simulink model "topcenterdown"  (Simulink 7.7)
settings: Solver=ode45  StartTime=0.0  StopTime=10.0  RelTol=1e-3
settings Model: Creator=Jx  LastModifiedBy=Jx

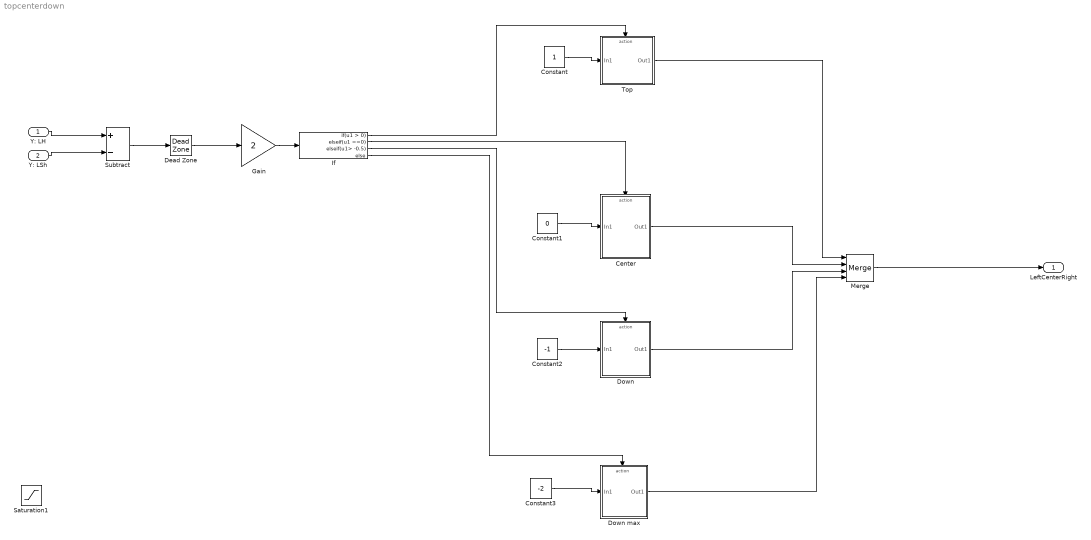
== system topcenterdown ==
  Y: LH : Inport
  Y: LSh : Inport  Port=2
  Center : Subsystem  TreatAsAtomicUnit=on
  Constant : Constant
  Constant1 : Constant  Value=0
  Constant2 : Constant  Value=-1
  Constant3 : Constant  Value=-2
  Dead Zone : DeadZone  LowerValue=-0.12  UpperValue=0.12  SaturateOnIntegerOverflow=on
  Down : Subsystem  TreatAsAtomicUnit=on
  Down max : Subsystem  TreatAsAtomicUnit=on
  Gain : Gain  Gain=2
  If : If  ElseIfExpressions=u1 ==0, u1> -0.5
  Merge : Merge  Inputs=4
  Saturation1 : Saturate  UpperLimit=1  LowerLimit=-1
  Subtract : Sum  Inputs=+-
  Top : Subsystem  TreatAsAtomicUnit=on
  LeftCenterRight : Outport
  wires:
  Y: LSh/1 -> Subtract/2
  Y: LH/1 -> Subtract/1
  Subtract/1 -> Dead Zone/1
  If/1 -> Top/Action
  If/2 -> Center/Action
  If/3 -> Down/Action
  If/4 -> Down max/Action
  Constant/1 -> Top/1(In1)
  Dead Zone/1 -> Gain/1
  Gain/1 -> If/1
  Constant1/1 -> Center/1(In1)
  Constant2/1 -> Down/1(In1)
  Constant3/1 -> Down max/1(In1)
  Center/1(Out1) -> Merge/2
  Down/1(Out1) -> Merge/3
  Down max/1(Out1) -> Merge/4
  Top/1(Out1) -> Merge/1
  Merge/1 -> LeftCenterRight/1

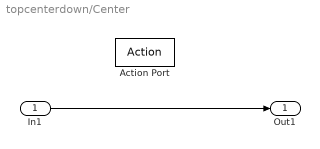
== system topcenterdown/Center ==
  In1 : Inport
  Action Port : ActionPort  ActionType=elseif
  Out1 : Outport
  wires:
  In1/1 -> Out1/1

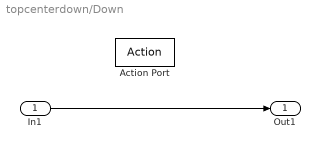
== system topcenterdown/Down ==
  In1 : Inport
  Action Port : ActionPort  ActionType=elseif
  Out1 : Outport
  wires:
  In1/1 -> Out1/1

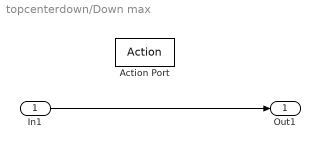
== system topcenterdown/Down max ==
  In1 : Inport
  Action Port : ActionPort  ActionType=else
  Out1 : Outport
  wires:
  In1/1 -> Out1/1

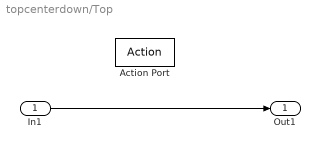
== system topcenterdown/Top ==
  In1 : Inport
  Action Port : ActionPort  ActionType=then
  Out1 : Outport
  wires:
  In1/1 -> Out1/1
